simulink model "CF017A_GmVehPwrMod"  (R2013b)
settings: Solver=FixedStepDiscrete  SolverMode=SingleTasking  StartTime=0.0  StopTime=2  FixedStep=0.002  RelTol=1e-3
values from neighbouring files (symbols this model uses):
  ASSIKEEPMINIDX_CNT_U16 = DataDict.Constant    [CF017A_GmVehPwrMod_DataDict.m]
  BUSOFFHISPDIDX_CNT_U16 = DataDict.Constant    [CF017A_GmVehPwrMod_DataDict.m]
  CNTTOSEC_ULS_U32 = DataDict.Constant    [CF017A_GmVehPwrMod_DataDict.m]
  ENGRUNACTVIDX_CNT_U16 = DataDict.Constant    [CF017A_GmVehPwrMod_DataDict.m]
  GmVehPwrModHwTqMinKeepAssi = DataDict.Calibration    [CF017A_GmVehPwrMod_DataDict.m]
  GmVehPwrModHwTqMinKeepTmr = DataDict.Calibration    [CF017A_GmVehPwrMod_DataDict.m]
  GmVehPwrModOperRampRate = DataDict.Calibration    [CF017A_GmVehPwrMod_DataDict.m]
  GMVEHPWRMODSYSSTREQENA_CNT_LOGL = DataDict.Constant    [CF017A_GmVehPwrMod_DataDict.m]
  GMVEHPWRMODVAREFF_CNT_LOGL = DataDict.Constant    [CF017A_GmVehPwrMod_DataDict.m]
  GmVehPwrModVehSpdAssiOnMin = DataDict.Calibration    [CF017A_GmVehPwrMod_DataDict.m]
  GmVehPwrModVehSpdMinKeepAssi = DataDict.Calibration    [CF017A_GmVehPwrMod_DataDict.m]
  GPIOMCUENAIDX_CNT_U16 = DataDict.Constant    [CF017A_GmVehPwrMod_DataDict.m]
  KEEPASSIIDX_CNT_U16 = DataDict.Constant    [CF017A_GmVehPwrMod_DataDict.m]
  MSG0C9MISSIDX_CNT_U16 = DataDict.Constant    [CF017A_GmVehPwrMod_DataDict.m]
  MSG1F1MISSIDX_CNT_U16 = DataDict.Constant    [CF017A_GmVehPwrMod_DataDict.m]
  SYSPWRMODRUNIDX_CNT_U16 = DataDict.Constant    [CF017A_GmVehPwrMod_DataDict.m]
  VEHSPDSNSRVLDIDX_CNT_U16 = DataDict.Constant    [CF017A_GmVehPwrMod_DataDict.m]
libraries: simulink x2, NxtrLim x2, NxtrAbslt x1
(part 2 of 4)

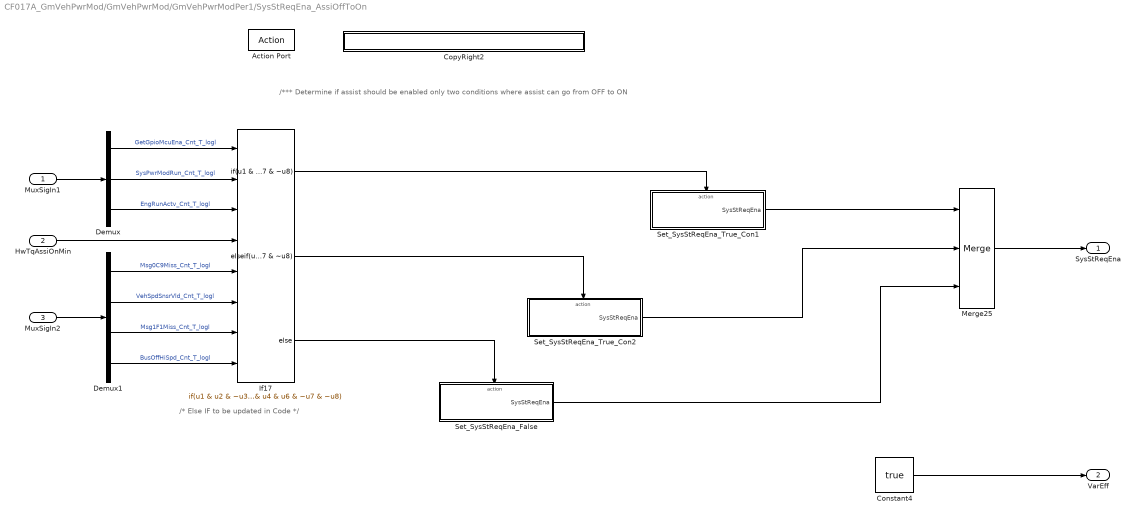
== system CF017A_GmVehPwrMod/GmVehPwrMod/GmVehPwrModPer1/SysStReqEna_AssiOffToOn ==
  note: /*** Determine if assist should be enabled only two conditions where assist can go from OFF to ON
  note: /* Else IF to be updated in Code */
  MuxSigIn1 : Inport  RequirementInfo="{'linktype_rmi_doors' '0000c6e5 (/GM T1XX/SubSystem Specifications/Customer Functions/CF017A GM Vehicle Power Mode)' '#CF017A_130' 'true' 'REQ:  CF017A_130' '' ; 'linktype_rmi_doors' '0000c6e5 (/GM T1XX/SubSystem Specifications/Customer Functions/CF017A GM Vehicle Power Mode)' '#CF017A_132' 'true' 'REQ:  CF017A_132' '' } %GIDa_3a645f64_a298_4f67_994e_ae497c860913"  OutDataTypeStr=boolean
  HwTqAssiOnMin : Inport  RequirementInfo="{'linktype_rmi_doors' '0000c6e5 (/GM T1XX/SubSystem Specifications/Customer Functions/CF017A GM Vehicle Power Mode)' '#CF017A_130' 'true' 'REQ:  CF017A_130' '' ; 'linktype_rmi_doors' '0000c6e5 (/GM T1XX/SubSystem Specifications/Customer Functions/CF017A GM Vehicle Power Mode)' '#CF017A_132' 'true' 'REQ:  CF017A_132' '' } %GIDa_13b583ed_e90a_4416_8c30_10328e753036"  Port=2  OutDataTypeStr=boolean
  MuxSigIn2 : Inport  RequirementInfo="{'linktype_rmi_doors' '0000c6e5 (/GM T1XX/SubSystem Specifications/Customer Functions/CF017A GM Vehicle Power Mode)' '#CF017A_130' 'true' 'REQ:  CF017A_130' '' ; 'linktype_rmi_doors' '0000c6e5 (/GM T1XX/SubSystem Specifications/Customer Functions/CF017A GM Vehicle Power Mode)' '#CF017A_132' 'true' 'REQ:  CF017A_132' '' } %GIDa_8c575e92_6a15_4759_8faa_7f2f79c8bcbf"  Port=3  OutDataTypeStr=boolean
  Action Port : ActionPort  ActionType=elseif
  Constant4 : Constant  RequirementInfo="{'linktype_rmi_doors' '0000c6e5 (/GM T1XX/SubSystem Specifications/Customer Functions/CF017A GM Vehicle Power Mode)' '#CF017A_130' 'true' 'REQ:  CF017A_130' '' ; 'linktype_rmi_doors' '0000c6e5 (/GM T1XX/SubSystem Specifications/Customer Functions/CF017A GM Vehicle Power Mode)' '#CF017A_132' 'true' 'REQ:  CF017A_132' '' } %GIDa_28018b21_20e3_4540_86d7_d93f0b461aa2"  Value=true  OutDataTypeStr=boolean
      settings: AttributesFormatString=%<OutDataTypeStr>
  CopyRight2 : Subsystem  Description=|  mask(Copyright Information){none=on}
      | Copyright info block.                                               
      |                                                                     
      | Place copyright information at the top of every subsystem in design.
      mask prompts: none "No parameters"
      mask help: Place copyright information at the top of every subsystem in design.
      mask Display:
      | NxtrConf = 'Nexteer Confidential';
      | 
      | sys = bdroot; %handle for the current model ("system")
      | first = get_param(sys,'Created');
      | if(isempty(first))
      |     first = datestr(now,'yyyy');
      | else
      |     first = first(end-3:end);  %year is last four digits
      | end
      | 
      | last = get_param(sys,'LastModifiedDate');
      | if isempty(last)
      |     last = datestr(now,'yyyy');
      | else
      |     last = last(end-3:end);
      | end
      | 
      | if strcmp(first,last)
      |     fprintf('%s -- Copyright %s Nexteer',NxtrConf,first)
      | else
      |     fprintf('%s -- %s%s- %s Nexteer',NxtrConf,char(169),first,last)
      | end
  Demux : Demux  RequirementInfo="{'linktype_rmi_doors' '0000c6e5 (/GM T1XX/SubSystem Specifications/Customer Functions/CF017A GM Vehicle Power Mode)' '#CF017A_130' 'true' 'REQ:  CF017A_130' '' ; 'linktype_rmi_doors' '0000c6e5 (/GM T1XX/SubSystem Specifications/Customer Functions/CF017A GM Vehicle Power Mode)' '#CF017A_132' 'true' 'REQ:  CF017A_132' '' } %GIDa_c957861a_4896_4335_9688_d9e475086b66"  Outputs=3
  Demux1 : Demux  RequirementInfo="{'linktype_rmi_doors' '0000c6e5 (/GM T1XX/SubSystem Specifications/Customer Functions/CF017A GM Vehicle Power Mode)' '#CF017A_130' 'true' 'REQ:  CF017A_130' '' ; 'linktype_rmi_doors' '0000c6e5 (/GM T1XX/SubSystem Specifications/Customer Functions/CF017A GM Vehicle Power Mode)' '#CF017A_132' 'true' 'REQ:  CF017A_132' '' } %GIDa_ca90b68c_293b_4a39_a1cb_c821dbb0cfb0"
  If17 : If  RequirementInfo="{'linktype_rmi_doors' '0000c6e5 (/GM T1XX/SubSystem Specifications/Customer Functions/CF017A GM Vehicle Power Mode)' '#CF017A_130' 'true' 'REQ:  CF017A_130' '' ; 'linktype_rmi_doors' '0000c6e5 (/GM T1XX/SubSystem Specifications/Customer Functions/CF017A GM Vehicle Power Mode)' '#CF017A_132' 'true' 'REQ:  CF017A_132' '' } %GIDa_e4b0cffb_9e91_44be_9216_eb129f9e2671"  NumInputs=8  IfExpression=u1 & u2 & ~u3 & u4 & u6 & ~u7 & ~u8  ElseIfExpressions=u1 & u2 & u3 & ~u5 & ~u7 & ~u8
      settings: AttributesFormatString=|
      | IF: %<IfExpression>
      | ElseIF: %<ElseIfExpressions>
  Merge25 : Merge  RequirementInfo="{'linktype_rmi_doors' '0000c6e5 (/GM T1XX/SubSystem Specifications/Customer Functions/CF017A GM Vehicle Power Mode)' '#CF017A_130' 'true' 'REQ:  CF017A_130' '' ; 'linktype_rmi_doors' '0000c6e5 (/GM T1XX/SubSystem Specifications/Customer Functions/CF017A GM Vehicle Power Mode)' '#CF017A_132' 'true' 'REQ:  CF017A_132' '' } %GIDa_219fe9d4_ea4b_4cc3_b7ae_583a3cf7ad0b"  Inputs=3
  Set_SysStReqEna_False : Subsystem  RequirementInfo="{'linktype_rmi_doors' '0000c6e5 (/GM T1XX/SubSystem Specifications/Customer Functions/CF017A GM Vehicle Power Mode)' '#CF017A_130' 'true' 'REQ:  CF017A_130' '' ; 'linktype_rmi_doors' '0000c6e5 (/GM T1XX/SubSystem Specifications/Customer Functions/CF017A GM Vehicle Power Mode)' '#CF017A_132' 'true' 'REQ:  CF017A_132' '' } %GIDa_3ca735ee_cf0b_4463_bd71_cb4947717510"  TreatAsAtomicUnit=on
  Set_SysStReqEna_True_Con1 : Subsystem  RequirementInfo="{'linktype_rmi_doors' '0000c6e5 (/GM T1XX/SubSystem Specifications/Customer Functions/CF017A GM Vehicle Power Mode)' '#CF017A_130' 'true' 'REQ:  CF017A_130' '' ; 'linktype_rmi_doors' '0000c6e5 (/GM T1XX/SubSystem Specifications/Customer Functions/CF017A GM Vehicle Power Mode)' '#CF017A_132' 'true' 'REQ:  CF017A_132' '' } %GIDa_60646708_95df_4ddf_8c50_fe37dba6062c"  TreatAsAtomicUnit=on
  Set_SysStReqEna_True_Con2 : Subsystem  RequirementInfo="{'linktype_rmi_doors' '0000c6e5 (/GM T1XX/SubSystem Specifications/Customer Functions/CF017A GM Vehicle Power Mode)' '#CF017A_130' 'true' 'REQ:  CF017A_130' '' ; 'linktype_rmi_doors' '0000c6e5 (/GM T1XX/SubSystem Specifications/Customer Functions/CF017A GM Vehicle Power Mode)' '#CF017A_132' 'true' 'REQ:  CF017A_132' '' } %GIDa_e217ae54_3c8e_4f5f_af2d_8865989b832c"  TreatAsAtomicUnit=on
  "SysStReqEna " : Outport  RequirementInfo="{'linktype_rmi_doors' '0000c6e5 (/GM T1XX/SubSystem Specifications/Customer Functions/CF017A GM Vehicle Power Mode)' '#CF017A_130' 'true' 'REQ:  CF017A_130' '' ; 'linktype_rmi_doors' '0000c6e5 (/GM T1XX/SubSystem Specifications/Customer Functions/CF017A GM Vehicle Power Mode)' '#CF017A_132' 'true' 'REQ:  CF017A_132' '' } %GIDa_fc4160b3_c37f_4374_9d60_d4a4461d5e5a"
  "VarEff " : Outport  RequirementInfo="{'linktype_rmi_doors' '0000c6e5 (/GM T1XX/SubSystem Specifications/Customer Functions/CF017A GM Vehicle Power Mode)' '#CF017A_130' 'true' 'REQ:  CF017A_130' '' ; 'linktype_rmi_doors' '0000c6e5 (/GM T1XX/SubSystem Specifications/Customer Functions/CF017A GM Vehicle Power Mode)' '#CF017A_132' 'true' 'REQ:  CF017A_132' '' } %GIDa_0e96ca85_c5e8_49ff_8347_73e0e2c63760"  Port=2
  wires:
  If17/1 -> Set_SysStReqEna_True_Con1/Action
  If17/2 -> Set_SysStReqEna_True_Con2/Action
  If17/3 -> Set_SysStReqEna_False/Action
  Set_SysStReqEna_True_Con1/1(SysStReqEna) -> Merge25/1
  Set_SysStReqEna_True_Con2/1(SysStReqEna) -> Merge25/2
  HwTqAssiOnMin/1 -> If17/4
  Set_SysStReqEna_False/1(SysStReqEna) -> Merge25/3
  Merge25/1 -> "SysStReqEna "/1
  Demux/1 -> If17/1  "GetGpioMcuEna_Cnt_T_logl"
  Demux/2 -> If17/2  "SysPwrModRun_Cnt_T_logl"
  Demux/3 -> If17/3  "EngRunActv_Cnt_T_logl"
  Demux1/2 -> If17/6  "VehSpdSnsrVld_Cnt_T_logl"
  Demux1/1 -> If17/5  "Msg0C9Miss_Cnt_T_logl"
  Demux1/3 -> If17/7  "Msg1F1Miss_Cnt_T_logl"
  Demux1/4 -> If17/8  "BusOffHiSpd_Cnt_T_logl"
  MuxSigIn2/1 -> Demux1/1
  MuxSigIn1/1 -> Demux/1
  Constant4/1 -> "VarEff "/1

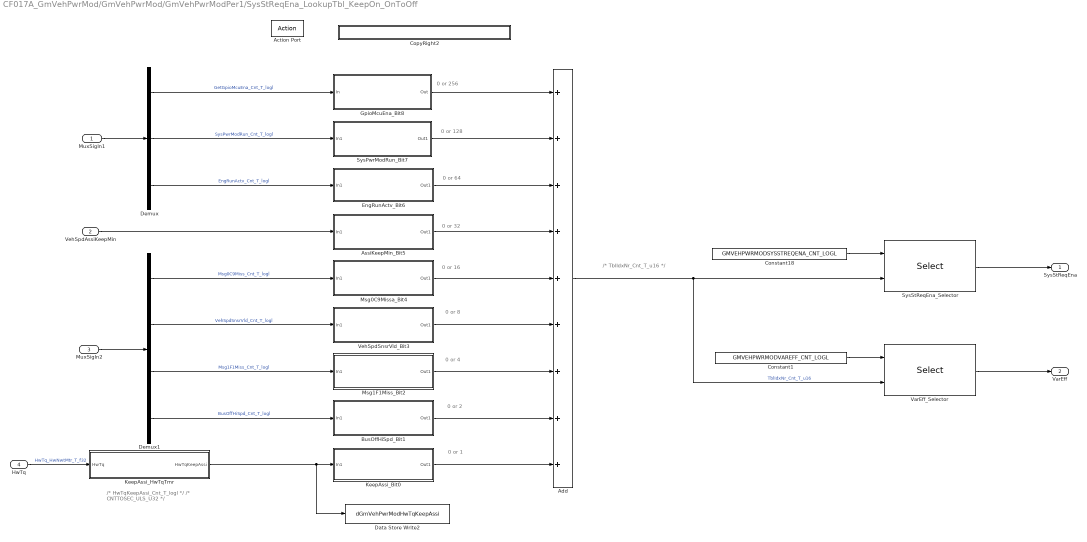
== system CF017A_GmVehPwrMod/GmVehPwrMod/GmVehPwrModPer1/SysStReqEna_LookupTbl_KeepOn_OnToOff ==
  note: 0 or 16
  note: 0 or 64
  note: 0 or 128
  note: 0 or 256
  note: 0 or 8
  note: 0 or 4
  note: 0 or 2
  note: 0 or 1
  note: 0 or 32
  note: /* TblIdxNr_Cnt_T_u16 */
  note: /* HwTqKeepAssi_Cnt_T_logl */
      | /* CNTTOSEC_ULS_U32 */
  MuxSigIn1 : Inport  RequirementInfo="{'linktype_rmi_doors' '0000c6e5 (/GM T1XX/SubSystem Specifications/Customer Functions/CF017A GM Vehicle Power Mode)' '#CF017A_114' 'true' 'REQ:  CF017A_114' '' } %GIDa_bc80a4e1_b6bc_4c53_b492_9b7a6973627c"  OutDataTypeStr=boolean
  VehSpdAssiKeepMin : Inport  RequirementInfo="{'linktype_rmi_doors' '0000c6e5 (/GM T1XX/SubSystem Specifications/Customer Functions/CF017A GM Vehicle Power Mode)' '#CF017A_114' 'true' 'REQ:  CF017A_114' '' } %GIDa_6ee4d72d_68c9_4a05_8ea5_3d3973aae7e5"  Port=2
  MuxSigIn2 : Inport  RequirementInfo="{'linktype_rmi_doors' '0000c6e5 (/GM T1XX/SubSystem Specifications/Customer Functions/CF017A GM Vehicle Power Mode)' '#CF017A_114' 'true' 'REQ:  CF017A_114' '' } %GIDa_08dc748f_4306_4e77_85d5_d7c5491b97dc"  Port=3  OutDataTypeStr=boolean
  HwTq : Inport  RequirementInfo="{'linktype_rmi_doors' '0000c6e5 (/GM T1XX/SubSystem Specifications/Customer Functions/CF017A GM Vehicle Power Mode)' '#CF017A_114' 'true' 'REQ:  CF017A_114' '' } %GIDa_7ab02a14_6014_485c_9516_71370e70d1f4"  Port=4
  Action Port : ActionPort  ActionType=else
  Add : Sum  RequirementInfo="{'linktype_rmi_doors' '0000c6e5 (/GM T1XX/SubSystem Specifications/Customer Functions/CF017A GM Vehicle Power Mode)' '#CF017A_114' 'true' 'REQ:  CF017A_114' '' } %GIDa_af12cd49_a835_4f7e_b3ef_f6819d7b005a"  Inputs=+++++++++
  AssiKeepMin_Bit5 : Subsystem  RequirementInfo="{'linktype_rmi_doors' '0000c6e5 (/GM T1XX/SubSystem Specifications/Customer Functions/CF017A GM Vehicle Power Mode)' '#CF017A_114' 'true' 'REQ:  CF017A_114' '' } %GIDa_94f80c15_8d5b_4603_bc32_7f6308c62976"
  BusOffHiSpd_Bit1 : Subsystem  RequirementInfo="{'linktype_rmi_doors' '0000c6e5 (/GM T1XX/SubSystem Specifications/Customer Functions/CF017A GM Vehicle Power Mode)' '#CF017A_114' 'true' 'REQ:  CF017A_114' '' } %GIDa_acd920ac_0f8e_48b1_8cb3_47da6f21ab97"
  Constant1 : Constant  RequirementInfo="{'linktype_rmi_doors' '0000c6e5 (/GM T1XX/SubSystem Specifications/Customer Functions/CF017A GM Vehicle Power Mode)' '#CF017A_114' 'true' 'REQ:  CF017A_114' '' } %GIDa_f83ca8bd_5e56_4e06_a072_f0a295a990ca"  Value=GMVEHPWRMODVAREFF_CNT_LOGL
  Constant18 : Constant  RequirementInfo="{'linktype_rmi_doors' '0000c6e5 (/GM T1XX/SubSystem Specifications/Customer Functions/CF017A GM Vehicle Power Mode)' '#CF017A_114' 'true' 'REQ:  CF017A_114' '' } %GIDa_ed68045e_dae1_4310_b1cc_3761b5a41fc7"  Value=GMVEHPWRMODSYSSTREQENA_CNT_LOGL
  CopyRight2 : Subsystem  Description=|  mask(Copyright Information){none=on}
      | Copyright info block.                                               
      |                                                                     
      | Place copyright information at the top of every subsystem in design.
      mask prompts: none "No parameters"
      mask help: Place copyright information at the top of every subsystem in design.
      mask Display:
      | NxtrConf = 'Nexteer Confidential';
      | 
      | sys = bdroot; %handle for the current model ("system")
      | first = get_param(sys,'Created');
      | if(isempty(first))
      |     first = datestr(now,'yyyy');
      | else
      |     first = first(end-3:end);  %year is last four digits
      | end
      | 
      | last = get_param(sys,'LastModifiedDate');
      | if isempty(last)
      |     last = datestr(now,'yyyy');
      | else
      |     last = last(end-3:end);
      | end
      | 
      | if strcmp(first,last)
      |     fprintf('%s -- Copyright %s Nexteer',NxtrConf,first)
      | else
      |     fprintf('%s -- %s%s- %s Nexteer',NxtrConf,char(169),first,last)
      | end
  Data Store Write2 : DataStoreWrite  DataStoreName=dGmVehPwrModHwTqKeepAssi
  Demux : Demux  RequirementInfo="{'linktype_rmi_doors' '0000c6e5 (/GM T1XX/SubSystem Specifications/Customer Functions/CF017A GM Vehicle Power Mode)' '#CF017A_114' 'true' 'REQ:  CF017A_114' '' } %GIDa_88d4c8c0_301e_4e56_88eb_14518dbfa869"  Outputs=3
  Demux1 : Demux  RequirementInfo="{'linktype_rmi_doors' '0000c6e5 (/GM T1XX/SubSystem Specifications/Customer Functions/CF017A GM Vehicle Power Mode)' '#CF017A_114' 'true' 'REQ:  CF017A_114' '' } %GIDa_f49741f0_2463_44a9_89b1_7362f5f0fc1c"
  EngRunActv_Bit6 : Subsystem  RequirementInfo="{'linktype_rmi_doors' '0000c6e5 (/GM T1XX/SubSystem Specifications/Customer Functions/CF017A GM Vehicle Power Mode)' '#CF017A_114' 'true' 'REQ:  CF017A_114' '' } %GIDa_75e4a1a1_cdfd_4aa7_88fa_f6563dcb65b2"
  GpioMcuEna_Bit8 : Subsystem  RequirementInfo="{'linktype_rmi_doors' '0000c6e5 (/GM T1XX/SubSystem Specifications/Customer Functions/CF017A GM Vehicle Power Mode)' '#CF017A_114' 'true' 'REQ:  CF017A_114' '' } %GIDa_beb8bd3a_ac5d_4344_8c2b_8f2faf648cc5"
  KeepAssi_Bit0 : Subsystem  RequirementInfo="{'linktype_rmi_doors' '0000c6e5 (/GM T1XX/SubSystem Specifications/Customer Functions/CF017A GM Vehicle Power Mode)' '#CF017A_114' 'true' 'REQ:  CF017A_114' '' } %GIDa_b6564b7a_9176_438f_bd2a_268c0898aa62"
  KeepAssi_HwTqTmr : Subsystem  RequirementInfo="{'linktype_rmi_doors' '0000c6e5 (/GM T1XX/SubSystem Specifications/Customer Functions/CF017A GM Vehicle Power Mode)' '#CF017A_114' 'true' 'REQ:  CF017A_114' '' } %GIDa_4a627334_04f0_4326_b091_1c280c9a11a7"
  Msg0C9Missa_Bit4 : Subsystem  RequirementInfo="{'linktype_rmi_doors' '0000c6e5 (/GM T1XX/SubSystem Specifications/Customer Functions/CF017A GM Vehicle Power Mode)' '#CF017A_114' 'true' 'REQ:  CF017A_114' '' } %GIDa_5b52aa49_2ebb_4a5b_8b41_64565aeaf0de"
  Msg1F1Miss_Bit2 : Subsystem  RequirementInfo="{'linktype_rmi_doors' '0000c6e5 (/GM T1XX/SubSystem Specifications/Customer Functions/CF017A GM Vehicle Power Mode)' '#CF017A_114' 'true' 'REQ:  CF017A_114' '' } %GIDa_0c41f67f_7314_48ed_b309_7584390071f0"
  SysPwrModRun_Bit7 : Subsystem  RequirementInfo="{'linktype_rmi_doors' '0000c6e5 (/GM T1XX/SubSystem Specifications/Customer Functions/CF017A GM Vehicle Power Mode)' '#CF017A_114' 'true' 'REQ:  CF017A_114' '' } %GIDa_84b4e559_e806_45d4_a3c5_9c7f1e52808b"
  SysStReqEna_Selector : Selector  RequirementInfo="{'linktype_rmi_doors' '0000c6e5 (/GM T1XX/SubSystem Specifications/Customer Functions/CF017A GM Vehicle Power Mode)' '#CF017A_114' 'true' 'REQ:  CF017A_114' '' } %GIDa_e2ec4604_e247_4eee_afce_2078a19115c9"  IndexMode=Zero-based  InputPortWidth=512  IndexOptions=Index vector (port)  Indices=[1 3]  OutputSizes=1
  VarEff_Selector : Selector  RequirementInfo="{'linktype_rmi_doors' '0000c6e5 (/GM T1XX/SubSystem Specifications/Customer Functions/CF017A GM Vehicle Power Mode)' '#CF017A_114' 'true' 'REQ:  CF017A_114' '' } %GIDa_e88c0b5b_7fa6_44e0_af9c_6c470f98259a"  IndexMode=Zero-based  InputPortWidth=512  IndexOptions=Index vector (port)  Indices=[1 3]  OutputSizes=1
  VehSpdSnsrVld_Bit3 : Subsystem  RequirementInfo="{'linktype_rmi_doors' '0000c6e5 (/GM T1XX/SubSystem Specifications/Customer Functions/CF017A GM Vehicle Power Mode)' '#CF017A_114' 'true' 'REQ:  CF017A_114' '' } %GIDa_ee67c329_461f_4602_8c3a_261f4dbd38de"
  "SysStReqEna " : Outport  RequirementInfo="{'linktype_rmi_doors' '0000c6e5 (/GM T1XX/SubSystem Specifications/Customer Functions/CF017A GM Vehicle Power Mode)' '#CF017A_114' 'true' 'REQ:  CF017A_114' '' } %GIDa_ff1809e7_8b99_40a3_9863_33421325c6cd"
  VarEff : Outport  RequirementInfo="{'linktype_rmi_doors' '0000c6e5 (/GM T1XX/SubSystem Specifications/Customer Functions/CF017A GM Vehicle Power Mode)' '#CF017A_114' 'true' 'REQ:  CF017A_114' '' } %GIDa_1c4d589a_3e48_4ee3_8a43_5aea24c8ecda"  Port=2
  wires:
  SysStReqEna_Selector/1 -> "SysStReqEna "/1
  Constant18/1 -> SysStReqEna_Selector/1
  VarEff_Selector/1 -> VarEff/1
  Constant1/1 -> VarEff_Selector/1
  MuxSigIn2/1 -> Demux1/1
  MuxSigIn1/1 -> Demux/1
  Add/1 -> SysStReqEna_Selector/2, VarEff_Selector/2  "TblIdxNr_Cnt_T_u16"
  HwTq/1 -> KeepAssi_HwTqTmr/1(HwTq)  "HwTq_HwNwtMtr_T_f32"
  Demux/1 -> GpioMcuEna_Bit8/1(In)  "GetGpioMcuEna_Cnt_T_logl"
  GpioMcuEna_Bit8/1(Out) -> Add/1
  Demux/2 -> SysPwrModRun_Bit7/1(In1)  "SysPwrModRun_Cnt_T_logl"
  SysPwrModRun_Bit7/1(Out1) -> Add/2
  Demux/3 -> EngRunActv_Bit6/1(In1)  "EngRunActv_Cnt_T_logl"
  EngRunActv_Bit6/1(Out1) -> Add/3
  VehSpdAssiKeepMin/1 -> AssiKeepMin_Bit5/1(In1)
  AssiKeepMin_Bit5/1(Out1) -> Add/4
  Demux1/1 -> Msg0C9Missa_Bit4/1(In1)  "Msg0C9Miss_Cnt_T_logl"
  Msg0C9Missa_Bit4/1(Out1) -> Add/5
  Demux1/2 -> VehSpdSnsrVld_Bit3/1(In1)  "VehSpdSnsrVld_Cnt_T_logl"
  VehSpdSnsrVld_Bit3/1(Out1) -> Add/6
  Demux1/3 -> Msg1F1Miss_Bit2/1(In1)  "Msg1F1Miss_Cnt_T_logl"
  Msg1F1Miss_Bit2/1(Out1) -> Add/7
  Demux1/4 -> BusOffHiSpd_Bit1/1(In1)  "BusOffHiSpd_Cnt_T_logl"
  BusOffHiSpd_Bit1/1(Out1) -> Add/8
  KeepAssi_HwTqTmr/1(HwTqKeepAssi) -> KeepAssi_Bit0/1(In1), Data Store Write2/1
  KeepAssi_Bit0/1(Out1) -> Add/9

== system CF017A_GmVehPwrMod/GmVehPwrMod/GmVehPwrModPer1/SysStReqEna_Ovrd ==
  Action Port : ActionPort  ActionType=then
  Constant1 : Constant  RequirementInfo={} %GIDa_86169540_2bc4_413c_97a3_0e1ca5ec957c  Value=true  OutDataTypeStr=boolean
      settings: AttributesFormatString=%<OutDataTypeStr>
  Constant4 : Constant  RequirementInfo="{'linktype_rmi_doors' '0000c6e5 (/GM T1XX/SubSystem Specifications/Customer Functions/CF017A GM Vehicle Power Mode)' '#CF017A_32' 'true' 'REQ:  CF017A_32' '' } %GIDa_c86d9dd6_1d05_446b_a018_9e405ef852b6"  Value=true  OutDataTypeStr=boolean
      settings: AttributesFormatString=%<OutDataTypeStr>
  CopyRight2 : Subsystem  Description=|  mask(Copyright Information){none=on}
      | Copyright info block.                                               
      |                                                                     
      | Place copyright information at the top of every subsystem in design.
      mask prompts: none "No parameters"
      mask help: Place copyright information at the top of every subsystem in design.
      mask Display:
      | NxtrConf = 'Nexteer Confidential';
      | 
      | sys = bdroot; %handle for the current model ("system")
      | first = get_param(sys,'Created');
      | if(isempty(first))
      |     first = datestr(now,'yyyy');
      | else
      |     first = first(end-3:end);  %year is last four digits
      | end
      | 
      | last = get_param(sys,'LastModifiedDate');
      | if isempty(last)
      |     last = datestr(now,'yyyy');
      | else
      |     last = last(end-3:end);
      | end
      | 
      | if strcmp(first,last)
      |     fprintf('%s -- Copyright %s Nexteer',NxtrConf,first)
      | else
      |     fprintf('%s -- %s%s- %s Nexteer',NxtrConf,char(169),first,last)
      | end
  "SysStReqEna " : Outport  RequirementInfo="{'linktype_rmi_doors' '0000c6e5 (/GM T1XX/SubSystem Specifications/Customer Functions/CF017A GM Vehicle Power Mode)' '#CF017A_32' 'true' 'REQ:  CF017A_32' '' } %GIDa_fef06345_7fe7_4764_9a7b_744e67a7009a"
  "VarEff " : Outport  RequirementInfo={} %GIDa_82925a69_3998_4825_a53d_8fd7debd7f3c  Port=2
  wires:
  Constant4/1 -> "SysStReqEna "/1
  Constant1/1 -> "VarEff "/1

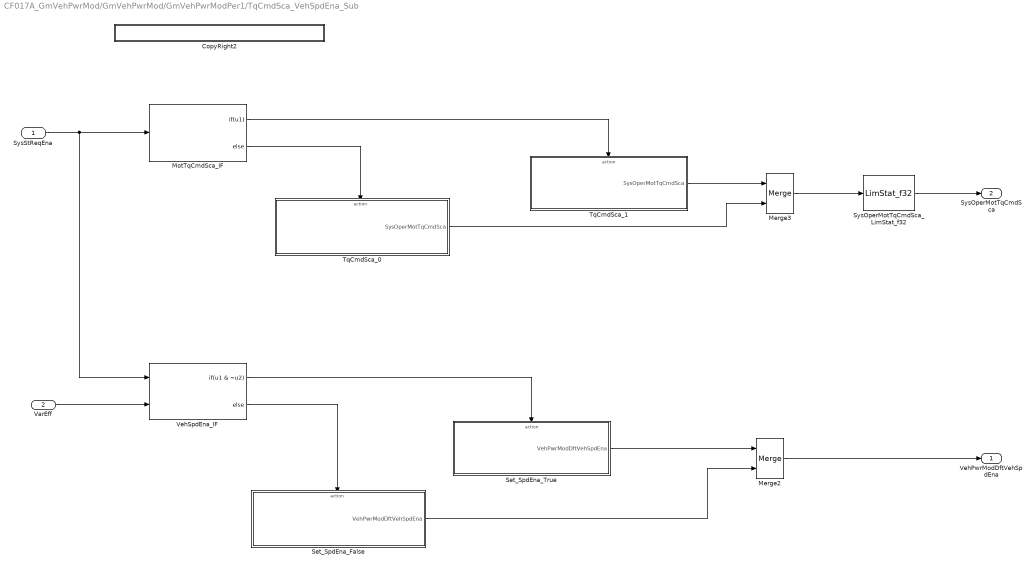
== system CF017A_GmVehPwrMod/GmVehPwrMod/GmVehPwrModPer1/TqCmdSca_VehSpdEna_Sub ==
  SysStReqEna : Inport  RequirementInfo="{'linktype_rmi_doors' '0000c6e5 (/GM T1XX/SubSystem Specifications/Customer Functions/CF017A GM Vehicle Power Mode)' '#CF017A_140' 'true' 'REQ:  CF017A_140' '' ; 'linktype_rmi_doors' '0000c6e5 (/GM T1XX/SubSystem Specifications/Customer Functions/CF017A GM Vehicle Power Mode)' '#CF017A_141' 'true' 'REQ:  CF017A_141' '' } %GIDa_01036905_94be_4768_a918_cd15c3b72ffe"
  VarEff : Inport  RequirementInfo="{'linktype_rmi_doors' '0000c6e5 (/GM T1XX/SubSystem Specifications/Customer Functions/CF017A GM Vehicle Power Mode)' '#CF017A_123' 'true' 'REQ:  CF017A_123' '' } %GIDa_07ed5c3a_8a5d_42c3_ba64_1b987a37fce0"  Port=2
  CopyRight2 : Subsystem  Description=|  mask(Copyright Information){none=on}
      | Copyright info block.                                               
      |                                                                     
      | Place copyright information at the top of every subsystem in design.
      mask prompts: none "No parameters"
      mask help: Place copyright information at the top of every subsystem in design.
      mask Display:
      | NxtrConf = 'Nexteer Confidential';
      | 
      | sys = bdroot; %handle for the current model ("system")
      | first = get_param(sys,'Created');
      | if(isempty(first))
      |     first = datestr(now,'yyyy');
      | else
      |     first = first(end-3:end);  %year is last four digits
      | end
      | 
      | last = get_param(sys,'LastModifiedDate');
      | if isempty(last)
      |     last = datestr(now,'yyyy');
      | else
      |     last = last(end-3:end);
      | end
      | 
      | if strcmp(first,last)
      |     fprintf('%s -- Copyright %s Nexteer',NxtrConf,first)
      | else
      |     fprintf('%s -- %s%s- %s Nexteer',NxtrConf,char(169),first,last)
      | end
  Merge2 : Merge  RequirementInfo="{'linktype_rmi_doors' '0000c6e5 (/GM T1XX/SubSystem Specifications/Customer Functions/CF017A GM Vehicle Power Mode)' '#CF017A_123' 'true' 'REQ:  CF017A_123' '' } %GIDa_cc0f1064_8083_4311_9dd5_460ed1fc79d1"
  Merge3 : Merge  RequirementInfo="{'linktype_rmi_doors' '0000c6e5 (/GM T1XX/SubSystem Specifications/Customer Functions/CF017A GM Vehicle Power Mode)' '#CF017A_140' 'true' 'REQ:  CF017A_140' '' ; 'linktype_rmi_doors' '0000c6e5 (/GM T1XX/SubSystem Specifications/Customer Functions/CF017A GM Vehicle Power Mode)' '#CF017A_141' 'true' 'REQ:  CF017A_141' '' } %GIDa_7104efbd_2360_454f_bb59_9e1f25f24a84"
  MotTqCmdSca_IF : If  RequirementInfo="{'linktype_rmi_doors' '0000c6e5 (/GM T1XX/SubSystem Specifications/Customer Functions/CF017A GM Vehicle Power Mode)' '#CF017A_140' 'true' 'REQ:  CF017A_140' '' ; 'linktype_rmi_doors' '0000c6e5 (/GM T1XX/SubSystem Specifications/Customer Functions/CF017A GM Vehicle Power Mode)' '#CF017A_141' 'true' 'REQ:  CF017A_141' '' } %GIDa_950fd77a_f254_4eed_8851_b62a8f7157ad"  IfExpression=u1
      settings: AttributesFormatString=%<Priority>
  Set_SpdEna_False : Subsystem  RequirementInfo="{'linktype_rmi_doors' '0000c6e5 (/GM T1XX/SubSystem Specifications/Customer Functions/CF017A GM Vehicle Power Mode)' '#CF017A_123' 'true' 'REQ:  CF017A_123' '' } %GIDa_4c636395_5f2d_4a89_adaf_f2e48d7bef4f"  TreatAsAtomicUnit=on
  Set_SpdEna_True : Subsystem  RequirementInfo="{'linktype_rmi_doors' '0000c6e5 (/GM T1XX/SubSystem Specifications/Customer Functions/CF017A GM Vehicle Power Mode)' '#CF017A_123' 'true' 'REQ:  CF017A_123' '' } %GIDa_737d3150_8a6b_413f_a7a3_869252337b59"  TreatAsAtomicUnit=on
  SysOperMotTqCmdSca_LimStat_f32 : NxtrLim/LimStat_f32  RequirementInfo="{'linktype_rmi_doors' '0000c6e5 (/GM T1XX/SubSystem Specifications/Customer Functions/CF017A GM Vehicle Power Mode)' '#CF017A_140' 'true' 'REQ:  CF017A_140' '' ; 'linktype_rmi_doors' '0000c6e5 (/GM T1XX/SubSystem Specifications/Customer Functions/CF017A GM Vehicle Power Mode)' '#CF017A_141' 'true' 'REQ:  CF017A_141' '' } %GIDa_4f9e7895_c7c7_41c2_9c8a_a053b7d9d264"  LoLim=MINMOTTQCMDSCA_ULS_F32  HiLim=MAXMOTTQCMDSCA_ULS_F32
      settings: AttributesFormatString=|
      | Low Limit: %<LoLim>
      | High Limit:%<HiLim>
  TqCmdSca_0 : Subsystem  RequirementInfo="{'linktype_rmi_doors' '0000c6e5 (/GM T1XX/SubSystem Specifications/Customer Functions/CF017A GM Vehicle Power Mode)' '#CF017A_141' 'true' 'REQ:  CF017A_141' '' } %GIDa_decad64b_52d2_4602_b339_eff7f5e3ed06"  TreatAsAtomicUnit=on
  TqCmdSca_1 : Subsystem  RequirementInfo="{'linktype_rmi_doors' '0000c6e5 (/GM T1XX/SubSystem Specifications/Customer Functions/CF017A GM Vehicle Power Mode)' '#CF017A_140' 'true' 'REQ:  CF017A_140' '' } %GIDa_694753cb_c62a_470b_957a_ceb5f623f085"  TreatAsAtomicUnit=on
  VehSpdEna_IF : If  RequirementInfo="{'linktype_rmi_doors' '0000c6e5 (/GM T1XX/SubSystem Specifications/Customer Functions/CF017A GM Vehicle Power Mode)' '#CF017A_123' 'true' 'REQ:  CF017A_123' '' } %GIDa_4131b3ca_d781_465d_8cb6_f16244f312e7"  NumInputs=2  IfExpression=u1 & ~u2
      settings: AttributesFormatString=%<Priority>
  VehPwrModDftVehSpdEna : Outport  RequirementInfo="{'linktype_rmi_doors' '0000c6e5 (/GM T1XX/SubSystem Specifications/Customer Functions/CF017A GM Vehicle Power Mode)' '#CF017A_123' 'true' 'REQ:  CF017A_123' '' } %GIDa_9f3ed68c_cc4b_4ea7_b1f1_e6ba382b3ffd"
  SysOperMotTqCmdSca : Outport  RequirementInfo="{'linktype_rmi_doors' '0000c6e5 (/GM T1XX/SubSystem Specifications/Customer Functions/CF017A GM Vehicle Power Mode)' '#CF017A_140' 'true' 'REQ:  CF017A_140' '' ; 'linktype_rmi_doors' '0000c6e5 (/GM T1XX/SubSystem Specifications/Customer Functions/CF017A GM Vehicle Power Mode)' '#CF017A_141' 'true' 'REQ:  CF017A_141' '' } %GIDa_e89f99b6_2659_40bd_8094_1ba8e8190b3a"  Port=2
  wires:
  Merge2/1 -> VehPwrModDftVehSpdEna/1
  VehSpdEna_IF/1 -> Set_SpdEna_True/Action
  Set_SpdEna_True/1("VehPwrModDftVehSpdEna ") -> Merge2/1
  VehSpdEna_IF/2 -> Set_SpdEna_False/Action
  Set_SpdEna_False/1("VehPwrModDftVehSpdEna ") -> Merge2/2
  VarEff/1 -> VehSpdEna_IF/2
  SysOperMotTqCmdSca_LimStat_f32/1 -> SysOperMotTqCmdSca/1
  Merge3/1 -> SysOperMotTqCmdSca_LimStat_f32/1
  SysStReqEna/1 -> VehSpdEna_IF/1, MotTqCmdSca_IF/1
  MotTqCmdSca_IF/1 -> TqCmdSca_1/Action
  MotTqCmdSca_IF/2 -> TqCmdSca_0/Action
  TqCmdSca_1/1(SysOperMotTqCmdSca) -> Merge3/1
  TqCmdSca_0/1(SysOperMotTqCmdSca) -> Merge3/2

== system CF017A_GmVehPwrMod/GmVehPwrMod/GmVehPwrModPer1/AssiOnMin_AssiKeepMin/AssiKeepMin_False ==
  Action Port : ActionPort  ActionType=else
  Constant4 : Constant  RequirementInfo={} %GIDa_c7fdf16e_9e64_43bf_82dd_e5311109beea  Value=false  OutDataTypeStr=boolean
      settings: AttributesFormatString=%<OutDataTypeStr>
  CopyRight2 : Subsystem  Description=|  mask(Copyright Information){none=on}
      | Copyright info block.                                               
      |                                                                     
      | Place copyright information at the top of every subsystem in design.
      mask prompts: none "No parameters"
      mask help: Place copyright information at the top of every subsystem in design.
      mask Display:
      | NxtrConf = 'Nexteer Confidential';
      | 
      | sys = bdroot; %handle for the current model ("system")
      | first = get_param(sys,'Created');
      | if(isempty(first))
      |     first = datestr(now,'yyyy');
      | else
      |     first = first(end-3:end);  %year is last four digits
      | end
      | 
      | last = get_param(sys,'LastModifiedDate');
      | if isempty(last)
      |     last = datestr(now,'yyyy');
      | else
      |     last = last(end-3:end);
      | end
      | 
      | if strcmp(first,last)
      |     fprintf('%s -- Copyright %s Nexteer',NxtrConf,first)
      | else
      |     fprintf('%s -- %s%s- %s Nexteer',NxtrConf,char(169),first,last)
      | end
  "AssiKeepMin " : Outport  RequirementInfo={} %GIDa_6901cb5a_957b_4373_94d3_bac0c9dabeaa
  wires:
  Constant4/1 -> "AssiKeepMin "/1

== system CF017A_GmVehPwrMod/GmVehPwrMod/GmVehPwrModPer1/AssiOnMin_AssiKeepMin/AssiKeepMin_True ==
  Action Port : ActionPort  ActionType=then
  Constant4 : Constant  RequirementInfo={} %GIDa_9490490c_6ae9_41b7_960c_89221b0e8a20  Value=true  OutDataTypeStr=boolean
      settings: AttributesFormatString=%<OutDataTypeStr>
  CopyRight2 : Subsystem  Description=|  mask(Copyright Information){none=on}
      | Copyright info block.                                               
      |                                                                     
      | Place copyright information at the top of every subsystem in design.
      mask prompts: none "No parameters"
      mask help: Place copyright information at the top of every subsystem in design.
      mask Display:
      | NxtrConf = 'Nexteer Confidential';
      | 
      | sys = bdroot; %handle for the current model ("system")
      | first = get_param(sys,'Created');
      | if(isempty(first))
      |     first = datestr(now,'yyyy');
      | else
      |     first = first(end-3:end);  %year is last four digits
      | end
      | 
      | last = get_param(sys,'LastModifiedDate');
      | if isempty(last)
      |     last = datestr(now,'yyyy');
      | else
      |     last = last(end-3:end);
      | end
      | 
      | if strcmp(first,last)
      |     fprintf('%s -- Copyright %s Nexteer',NxtrConf,first)
      | else
      |     fprintf('%s -- %s%s- %s Nexteer',NxtrConf,char(169),first,last)
      | end
  "AssiKeepMin " : Outport  RequirementInfo={} %GIDa_b41ba438_a4fe_44a5_9957_2297c1a0f856
  wires:
  Constant4/1 -> "AssiKeepMin "/1

== system CF017A_GmVehPwrMod/GmVehPwrMod/GmVehPwrModPer1/AssiOnMin_AssiKeepMin/AssiOnMin_False ==
  Action Port : ActionPort  ActionType=else
  Constant4 : Constant  RequirementInfo={} %GIDa_5e587e53_c67f_459d_920e_ac412b083272  Value=false  OutDataTypeStr=boolean
      settings: AttributesFormatString=%<OutDataTypeStr>
  CopyRight2 : Subsystem  Description=|  mask(Copyright Information){none=on}
      | Copyright info block.                                               
      |                                                                     
      | Place copyright information at the top of every subsystem in design.
      mask prompts: none "No parameters"
      mask help: Place copyright information at the top of every subsystem in design.
      mask Display:
      | NxtrConf = 'Nexteer Confidential';
      | 
      | sys = bdroot; %handle for the current model ("system")
      | first = get_param(sys,'Created');
      | if(isempty(first))
      |     first = datestr(now,'yyyy');
      | else
      |     first = first(end-3:end);  %year is last four digits
      | end
      | 
      | last = get_param(sys,'LastModifiedDate');
      | if isempty(last)
      |     last = datestr(now,'yyyy');
      | else
      |     last = last(end-3:end);
      | end
      | 
      | if strcmp(first,last)
      |     fprintf('%s -- Copyright %s Nexteer',NxtrConf,first)
      | else
      |     fprintf('%s -- %s%s- %s Nexteer',NxtrConf,char(169),first,last)
      | end
  "AssiOnMin " : Outport  RequirementInfo={} %GIDa_06e6b64a_b60d_4310_8675_e36109ef9cd4
  wires:
  Constant4/1 -> "AssiOnMin "/1

== system CF017A_GmVehPwrMod/GmVehPwrMod/GmVehPwrModPer1/AssiOnMin_AssiKeepMin/AssiOnMin_True ==
  Action Port : ActionPort  ActionType=then
  Constant4 : Constant  RequirementInfo={} %GIDa_f80019f1_30f3_49ae_9a8f_59acc09eeab3  Value=true  OutDataTypeStr=boolean
      settings: AttributesFormatString=%<OutDataTypeStr>
  CopyRight2 : Subsystem  Description=|  mask(Copyright Information){none=on}
      | Copyright info block.                                               
      |                                                                     
      | Place copyright information at the top of every subsystem in design.
      mask prompts: none "No parameters"
      mask help: Place copyright information at the top of every subsystem in design.
      mask Display:
      | NxtrConf = 'Nexteer Confidential';
      | 
      | sys = bdroot; %handle for the current model ("system")
      | first = get_param(sys,'Created');
      | if(isempty(first))
      |     first = datestr(now,'yyyy');
      | else
      |     first = first(end-3:end);  %year is last four digits
      | end
      | 
      | last = get_param(sys,'LastModifiedDate');
      | if isempty(last)
      |     last = datestr(now,'yyyy');
      | else
      |     last = last(end-3:end);
      | end
      | 
      | if strcmp(first,last)
      |     fprintf('%s -- Copyright %s Nexteer',NxtrConf,first)
      | else
      |     fprintf('%s -- %s%s- %s Nexteer',NxtrConf,char(169),first,last)
      | end
  "AssiOnMin " : Outport  RequirementInfo={} %GIDa_aae985c7_98fc_4fe2_9e33_fd60824e720f
  wires:
  Constant4/1 -> "AssiOnMin "/1

== system CF017A_GmVehPwrMod/GmVehPwrMod/GmVehPwrModPer1/AssiOnMin_AssiKeepMin/CopyRight2 ==

== system CF017A_GmVehPwrMod/GmVehPwrMod/GmVehPwrModPer1/GetGpioMcuEna/CopyRight2 ==

== system CF017A_GmVehPwrMod/GmVehPwrMod/GmVehPwrModPer1/PwrSplyEnaReq_Sub/CopyRight2 ==

== system CF017A_GmVehPwrMod/GmVehPwrMod/GmVehPwrModPer1/PwrSplyEnaReq_Sub/PwrSplyEnReq_False ==
  Action Port : ActionPort  ActionType=then
  Constant4 : Constant  RequirementInfo={} %GIDa_6bcf13cd_6bc6_446a_a6e7_6383ebebc93c  Value=false  OutDataTypeStr=boolean
      settings: AttributesFormatString=%<OutDataTypeStr>
  CopyRight2 : Subsystem  Description=|  mask(Copyright Information){none=on}
      | Copyright info block.                                               
      |                                                                     
      | Place copyright information at the top of every subsystem in design.
      mask prompts: none "No parameters"
      mask help: Place copyright information at the top of every subsystem in design.
      mask Display:
      | NxtrConf = 'Nexteer Confidential';
      | 
      | sys = bdroot; %handle for the current model ("system")
      | first = get_param(sys,'Created');
      | if(isempty(first))
      |     first = datestr(now,'yyyy');
      | else
      |     first = first(end-3:end);  %year is last four digits
      | end
      | 
      | last = get_param(sys,'LastModifiedDate');
      | if isempty(last)
      |     last = datestr(now,'yyyy');
      | else
      |     last = last(end-3:end);
      | end
      | 
      | if strcmp(first,last)
      |     fprintf('%s -- Copyright %s Nexteer',NxtrConf,first)
      | else
      |     fprintf('%s -- %s%s- %s Nexteer',NxtrConf,char(169),first,last)
      | end
  "VehPwrModDftVehSpdEna " : Outport  RequirementInfo={} %GIDa_72cc516b_829e_4c06_badb_b99c6418f51c
  wires:
  Constant4/1 -> "VehPwrModDftVehSpdEna "/1

== system CF017A_GmVehPwrMod/GmVehPwrMod/GmVehPwrModPer1/PwrSplyEnaReq_Sub/PwrSplyEnReq_True ==
  Action Port : ActionPort  ActionType=else
  Constant4 : Constant  RequirementInfo={} %GIDa_f6257761_f32f_49a6_9f73_75b94f86bd20  Value=true  OutDataTypeStr=boolean
      settings: AttributesFormatString=%<OutDataTypeStr>
  CopyRight2 : Subsystem  Description=|  mask(Copyright Information){none=on}
      | Copyright info block.                                               
      |                                                                     
      | Place copyright information at the top of every subsystem in design.
      mask prompts: none "No parameters"
      mask help: Place copyright information at the top of every subsystem in design.
      mask Display:
      | NxtrConf = 'Nexteer Confidential';
      | 
      | sys = bdroot; %handle for the current model ("system")
      | first = get_param(sys,'Created');
      | if(isempty(first))
      |     first = datestr(now,'yyyy');
      | else
      |     first = first(end-3:end);  %year is last four digits
      | end
      | 
      | last = get_param(sys,'LastModifiedDate');
      | if isempty(last)
      |     last = datestr(now,'yyyy');
      | else
      |     last = last(end-3:end);
      | end
      | 
      | if strcmp(first,last)
      |     fprintf('%s -- Copyright %s Nexteer',NxtrConf,first)
      | else
      |     fprintf('%s -- %s%s- %s Nexteer',NxtrConf,char(169),first,last)
      | end
  "VehPwrModDftVehSpdEna " : Outport  RequirementInfo={} %GIDa_b2592a36_5b30_49dc_998a_a6b760d5203e
  wires:
  Constant4/1 -> "VehPwrModDftVehSpdEna "/1

== system CF017A_GmVehPwrMod/GmVehPwrMod/GmVehPwrModPer1/SysStReqEna_AssiOffToOn/CopyRight2 ==

== system CF017A_GmVehPwrMod/GmVehPwrMod/GmVehPwrModPer1/SysStReqEna_AssiOffToOn/Set_SysStReqEna_False ==
  Action Port : ActionPort  ActionType=else
  Constant2 : Constant  RequirementInfo={} %GIDa_c553a8da_c905_4d87_9c6c_430af151d25e  Value=false  OutDataTypeStr=boolean
      settings: AttributesFormatString=%<OutDataTypeStr>
  CopyRight2 : Subsystem  Description=|  mask(Copyright Information){none=on}
      | Copyright info block.                                               
      |                                                                     
      | Place copyright information at the top of every subsystem in design.
      mask prompts: none "No parameters"
      mask help: Place copyright information at the top of every subsystem in design.
      mask Display:
      | NxtrConf = 'Nexteer Confidential';
      | 
      | sys = bdroot; %handle for the current model ("system")
      | first = get_param(sys,'Created');
      | if(isempty(first))
      |     first = datestr(now,'yyyy');
      | else
      |     first = first(end-3:end);  %year is last four digits
      | end
      | 
      | last = get_param(sys,'LastModifiedDate');
      | if isempty(last)
      |     last = datestr(now,'yyyy');
      | else
      |     last = last(end-3:end);
      | end
      | 
      | if strcmp(first,last)
      |     fprintf('%s -- Copyright %s Nexteer',NxtrConf,first)
      | else
      |     fprintf('%s -- %s%s- %s Nexteer',NxtrConf,char(169),first,last)
      | end
  SysStReqEna : Outport  RequirementInfo={} %GIDa_0afb345b_f296_4218_8c56_52561c59f1fd
  wires:
  Constant2/1 -> SysStReqEna/1

== system CF017A_GmVehPwrMod/GmVehPwrMod/GmVehPwrModPer1/SysStReqEna_AssiOffToOn/Set_SysStReqEna_True_Con1 ==
  Action Port : ActionPort  ActionType=then
  Constant2 : Constant  RequirementInfo={} %GIDa_8ac49ca2_7e24_414b_a2b5_e8b716d7f226  Value=true  OutDataTypeStr=boolean
      settings: AttributesFormatString=%<OutDataTypeStr>
  CopyRight2 : Subsystem  Description=|  mask(Copyright Information){none=on}
      | Copyright info block.                                               
      |                                                                     
      | Place copyright information at the top of every subsystem in design.
      mask prompts: none "No parameters"
      mask help: Place copyright information at the top of every subsystem in design.
      mask Display:
      | NxtrConf = 'Nexteer Confidential';
      | 
      | sys = bdroot; %handle for the current model ("system")
      | first = get_param(sys,'Created');
      | if(isempty(first))
      |     first = datestr(now,'yyyy');
      | else
      |     first = first(end-3:end);  %year is last four digits
      | end
      | 
      | last = get_param(sys,'LastModifiedDate');
      | if isempty(last)
      |     last = datestr(now,'yyyy');
      | else
      |     last = last(end-3:end);
      | end
      | 
      | if strcmp(first,last)
      |     fprintf('%s -- Copyright %s Nexteer',NxtrConf,first)
      | else
      |     fprintf('%s -- %s%s- %s Nexteer',NxtrConf,char(169),first,last)
      | end
  SysStReqEna : Outport  RequirementInfo={} %GIDa_4776be27_fcc3_4d90_b709_c30d43401c4d
  wires:
  Constant2/1 -> SysStReqEna/1

== system CF017A_GmVehPwrMod/GmVehPwrMod/GmVehPwrModPer1/SysStReqEna_AssiOffToOn/Set_SysStReqEna_True_Con2 ==
  Action Port : ActionPort  ActionType=elseif
  Constant2 : Constant  RequirementInfo={} %GIDa_3f3f42cc_2b6d_4365_a3cb_5f431e3d6f5b  Value=true  OutDataTypeStr=boolean
      settings: AttributesFormatString=%<OutDataTypeStr>
  CopyRight2 : Subsystem  Description=|  mask(Copyright Information){none=on}
      | Copyright info block.                                               
      |                                                                     
      | Place copyright information at the top of every subsystem in design.
      mask prompts: none "No parameters"
      mask help: Place copyright information at the top of every subsystem in design.
      mask Display:
      | NxtrConf = 'Nexteer Confidential';
      | 
      | sys = bdroot; %handle for the current model ("system")
      | first = get_param(sys,'Created');
      | if(isempty(first))
      |     first = datestr(now,'yyyy');
      | else
      |     first = first(end-3:end);  %year is last four digits
      | end
      | 
      | last = get_param(sys,'LastModifiedDate');
      | if isempty(last)
      |     last = datestr(now,'yyyy');
      | else
      |     last = last(end-3:end);
      | end
      | 
      | if strcmp(first,last)
      |     fprintf('%s -- Copyright %s Nexteer',NxtrConf,first)
      | else
      |     fprintf('%s -- %s%s- %s Nexteer',NxtrConf,char(169),first,last)
      | end
  SysStReqEna : Outport  RequirementInfo={} %GIDa_193cb312_dfce_42c9_b5cf_94697c7ae084
  wires:
  Constant2/1 -> SysStReqEna/1

== system CF017A_GmVehPwrMod/GmVehPwrMod/GmVehPwrModPer1/SysStReqEna_LookupTbl_KeepOn_OnToOff/AssiKeepMin_Bit5 ==
  In1 : Inport  RequirementInfo="{'linktype_rmi_doors' '0000c6e5 (/GM T1XX/SubSystem Specifications/Customer Functions/CF017A GM Vehicle Power Mode)' '#CF017A_114' 'true' 'REQ:  CF017A_114' '' } %GIDa_2d14ad53_1e41_43bd_9d52_9cfe50f04283"
  AssiKeepMin_IF : If  RequirementInfo="{'linktype_rmi_doors' '0000c6e5 (/GM T1XX/SubSystem Specifications/Customer Functions/CF017A GM Vehicle Power Mode)' '#CF017A_114' 'true' 'REQ:  CF017A_114' '' } %GIDa_69ed5737_6e11_4d15_b957_302060fb1464"  IfExpression=u1
  Bit5_0 : Subsystem  RequirementInfo="{'linktype_rmi_doors' '0000c6e5 (/GM T1XX/SubSystem Specifications/Customer Functions/CF017A GM Vehicle Power Mode)' '#CF017A_114' 'true' 'REQ:  CF017A_114' '' } %GIDa_248cc24c_28f6_49ca_9aa9_73cb9f966886"  TreatAsAtomicUnit=on
  Bit5_32 : Subsystem  RequirementInfo="{'linktype_rmi_doors' '0000c6e5 (/GM T1XX/SubSystem Specifications/Customer Functions/CF017A GM Vehicle Power Mode)' '#CF017A_114' 'true' 'REQ:  CF017A_114' '' } %GIDa_87bce6f0_a73b_4aa2_8b40_4ae9cc515bcd"  TreatAsAtomicUnit=on
  CopyRight2 : Subsystem  Description=|  mask(Copyright Information){none=on}
      | Copyright info block.                                               
      |                                                                     
      | Place copyright information at the top of every subsystem in design.
      mask prompts: none "No parameters"
      mask help: Place copyright information at the top of every subsystem in design.
      mask Display:
      | NxtrConf = 'Nexteer Confidential';
      | 
      | sys = bdroot; %handle for the current model ("system")
      | first = get_param(sys,'Created');
      | if(isempty(first))
      |     first = datestr(now,'yyyy');
      | else
      |     first = first(end-3:end);  %year is last four digits
      | end
      | 
      | last = get_param(sys,'LastModifiedDate');
      | if isempty(last)
      |     last = datestr(now,'yyyy');
      | else
      |     last = last(end-3:end);
      | end
      | 
      | if strcmp(first,last)
      |     fprintf('%s -- Copyright %s Nexteer',NxtrConf,first)
      | else
      |     fprintf('%s -- %s%s- %s Nexteer',NxtrConf,char(169),first,last)
      | end
  Merge3 : Merge  RequirementInfo="{'linktype_rmi_doors' '0000c6e5 (/GM T1XX/SubSystem Specifications/Customer Functions/CF017A GM Vehicle Power Mode)' '#CF017A_114' 'true' 'REQ:  CF017A_114' '' } %GIDa_623c38d0_7c7d_44e4_b1dd_4b971ca6385b"
  Out1 : Outport  RequirementInfo="{'linktype_rmi_doors' '0000c6e5 (/GM T1XX/SubSystem Specifications/Customer Functions/CF017A GM Vehicle Power Mode)' '#CF017A_114' 'true' 'REQ:  CF017A_114' '' } %GIDa_00b0a8dc_4f0d_4dce_bd85_2b01665ae9f5"
  wires:
  AssiKeepMin_IF/1 -> Bit5_32/Action
  AssiKeepMin_IF/2 -> Bit5_0/Action
  Bit5_32/1(Bit5Sts) -> Merge3/1
  Bit5_0/1(Bit5Sts) -> Merge3/2
  Merge3/1 -> Out1/1
  In1/1 -> AssiKeepMin_IF/1

== system CF017A_GmVehPwrMod/GmVehPwrMod/GmVehPwrModPer1/SysStReqEna_LookupTbl_KeepOn_OnToOff/BusOffHiSpd_Bit1 ==
  In1 : Inport  RequirementInfo="{'linktype_rmi_doors' '0000c6e5 (/GM T1XX/SubSystem Specifications/Customer Functions/CF017A GM Vehicle Power Mode)' '#CF017A_114' 'true' 'REQ:  CF017A_114' '' } %GIDa_6fc5c9f5_6b38_403e_a58b_8c0763600249"
  Bit1_0 : Subsystem  RequirementInfo="{'linktype_rmi_doors' '0000c6e5 (/GM T1XX/SubSystem Specifications/Customer Functions/CF017A GM Vehicle Power Mode)' '#CF017A_114' 'true' 'REQ:  CF017A_114' '' } %GIDa_3b15fed5_fc4f_41e3_8c4a_852c725d57c9"  TreatAsAtomicUnit=on
  Bit1_2 : Subsystem  RequirementInfo="{'linktype_rmi_doors' '0000c6e5 (/GM T1XX/SubSystem Specifications/Customer Functions/CF017A GM Vehicle Power Mode)' '#CF017A_114' 'true' 'REQ:  CF017A_114' '' } %GIDa_3b4db275_4f97_4f27_bf40_25b3c7ca69e8"  TreatAsAtomicUnit=on
  BusOffHiSpd_IF : If  RequirementInfo="{'linktype_rmi_doors' '0000c6e5 (/GM T1XX/SubSystem Specifications/Customer Functions/CF017A GM Vehicle Power Mode)' '#CF017A_114' 'true' 'REQ:  CF017A_114' '' } %GIDa_3c8c13db_cbd3_4fa8_ab73_795fe8ea1f92"  IfExpression=u1
  CopyRight2 : Subsystem  Description=|  mask(Copyright Information){none=on}
      | Copyright info block.                                               
      |                                                                     
      | Place copyright information at the top of every subsystem in design.
      mask prompts: none "No parameters"
      mask help: Place copyright information at the top of every subsystem in design.
      mask Display:
      | NxtrConf = 'Nexteer Confidential';
      | 
      | sys = bdroot; %handle for the current model ("system")
      | first = get_param(sys,'Created');
      | if(isempty(first))
      |     first = datestr(now,'yyyy');
      | else
      |     first = first(end-3:end);  %year is last four digits
      | end
      | 
      | last = get_param(sys,'LastModifiedDate');
      | if isempty(last)
      |     last = datestr(now,'yyyy');
      | else
      |     last = last(end-3:end);
      | end
      | 
      | if strcmp(first,last)
      |     fprintf('%s -- Copyright %s Nexteer',NxtrConf,first)
      | else
      |     fprintf('%s -- %s%s- %s Nexteer',NxtrConf,char(169),first,last)
      | end
  Merge7 : Merge  RequirementInfo="{'linktype_rmi_doors' '0000c6e5 (/GM T1XX/SubSystem Specifications/Customer Functions/CF017A GM Vehicle Power Mode)' '#CF017A_114' 'true' 'REQ:  CF017A_114' '' } %GIDa_e7ca4393_3a3d_4baf_8ccc_bea8ec8174f2"
  Out1 : Outport  RequirementInfo="{'linktype_rmi_doors' '0000c6e5 (/GM T1XX/SubSystem Specifications/Customer Functions/CF017A GM Vehicle Power Mode)' '#CF017A_114' 'true' 'REQ:  CF017A_114' '' } %GIDa_dceff7a4_b7b3_4426_8611_a5e36c9a31c4"
  wires:
  In1/1 -> BusOffHiSpd_IF/1
  BusOffHiSpd_IF/1 -> Bit1_2/Action
  BusOffHiSpd_IF/2 -> Bit1_0/Action
  Bit1_2/1(Bit1Sts) -> Merge7/1
  Bit1_0/1(Bit1Sts) -> Merge7/2
  Merge7/1 -> Out1/1

== system CF017A_GmVehPwrMod/GmVehPwrMod/GmVehPwrModPer1/SysStReqEna_LookupTbl_KeepOn_OnToOff/CopyRight2 ==
